simulink model "taratura_reazione_stato"  (R2025b)
settings: Solver=VariableStepAuto  StartTime=0.0  StopTime=30  RelTol=1e-3
undefined symbols (not defined in the file): dF_step_amp, dF_step_time, teta_zero, x_rif_step_amp, x_rif_step_time
settings Model: Creator=USER  LastModifiedBy=francesco
settings SolverCC: AlgebraicLoopSolver=TrustRegion
settings DebuggingCC: AlgebraicLoopMsg=none  UnconnectedInputMsg=warning  UnconnectedOutputMsg=warning  UnconnectedLineMsg=warning
settings ModelReferenceCC: EnableRefExpFcnMdlSchedulingChecks=on
settings RTWCC: GPUComputeCapability=3.5  DLArmComputeVersion=19.05

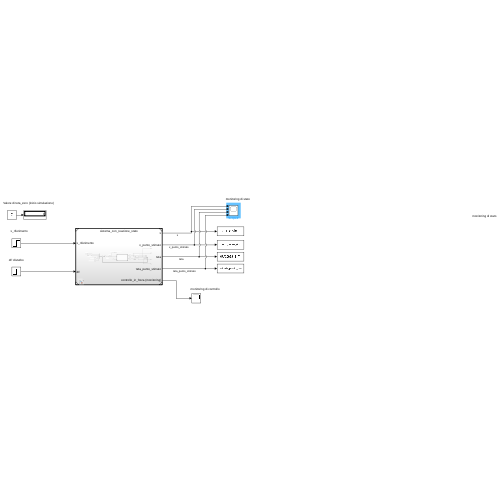
[thumbnail: Simulink's stored preview of the top-level diagram]
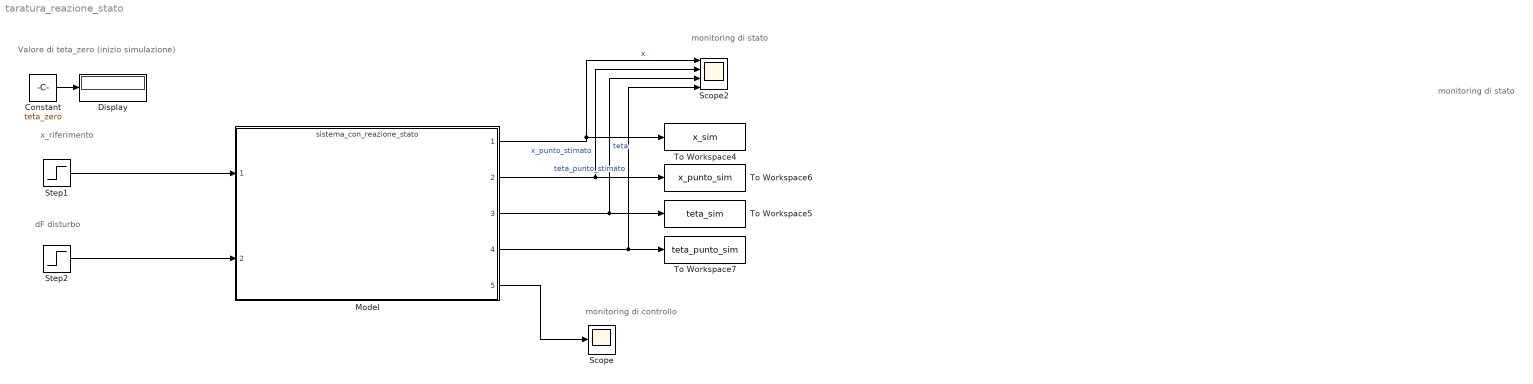
== system taratura_reazione_stato ==
  note: monitoring di controllo
  note: monitoring di stato
  note: x_riferimento
  note: Valore di teta_zero (inizio simulazione)
  note: monitoring di stato
  note: dF disturbo
  Constant : Constant  Value=teta_zero
  Display : Display
  Model : ModelReference  ModelNameDialog=sistema_con_reazione_stato.slx  SimulationMode=Normal  ModelReferenceVersion=9.54
  Scope : Scope
      settings: ActiveDisplayYMinimum=-1  ActiveDisplayYMaximum=1  DataLoggingVariableName=ScopeData2
  Scope2 : Scope  NumInputPorts=4
      settings: ActiveDisplayString=4  ActiveDisplayYMinimum=-0.11621866519085522  ActiveDisplayYMaximum=0.053248127870999085
      settings: ClipboardFcn=|
      | % eseguo la simulazione
      | simOut = sim('taratura_reazione_stato', 10); %10 secondi
  Step1 : Step  Time=x_rif_step_time  After=x_rif_step_amp  SampleTime=0
  Step2 : Step  Time=dF_step_time  After=dF_step_amp  SampleTime=0
  To Workspace4 : ToWorkspace  VariableName=x_sim  SaveFormat=Timeseries  SampleTime=-1
  To Workspace5 : ToWorkspace  VariableName=teta_sim  SaveFormat=Timeseries  SampleTime=-1
  To Workspace6 : ToWorkspace  VariableName=x_punto_sim  SaveFormat=Timeseries  SampleTime=-1
  To Workspace7 : ToWorkspace  VariableName=teta_punto_sim  SaveFormat=Timeseries  SampleTime=-1
  wires:
  Step1/1 -> Model/1
  Constant/1 -> Display/1
  Step2/1 -> Model/2
  Model/2 -> Scope2/2, To Workspace6/1  "x_punto_stimato"
  Model/1 -> To Workspace4/1, Scope2/1  "x"
  Model/3 -> To Workspace5/1, Scope2/3  "teta"
  Model/4 -> To Workspace7/1, Scope2/4  "teta_punto_stimato"
  Model/5 -> Scope/1
